simulink model "sampleModel1529"  (R2023a)
settings: Solver=VariableStepAuto  StartTime=0.0  StopTime=10.0  RelTol=1e-3
libraries: hdlsllib x6
settings Model: Creator=user1  LastModifiedBy=user1

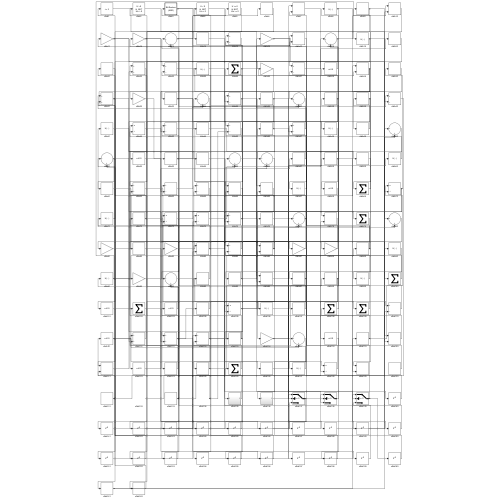
[thumbnail: Simulink's stored preview of the top-level diagram]
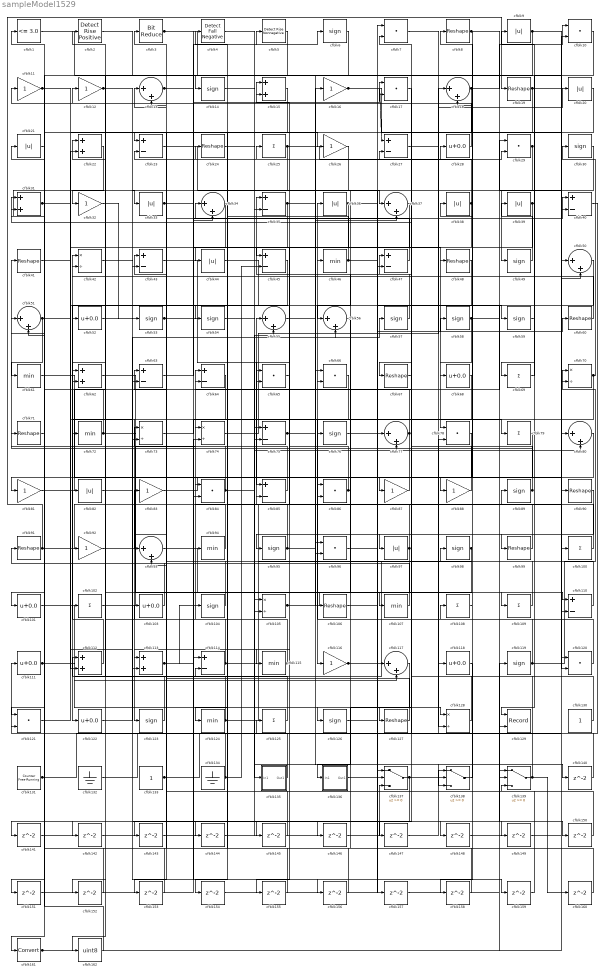
== system sampleModel1529 ==
  cfblk1 : hdlsllib/Logic and Bit Operations/Compare To Constant  relop=<=  const=3.0  OutDataTypeStr=boolean
  cfblk{7,10,17,29,65..66,78,84,86,96,120..121} (12 alike) : DotProduct  OutDataTypeStr=Inherit: Inherit via internal rule
  cfblk{25,69,79,100,102,108..109,125} (8 alike) : Sum  Inputs=+
  cfblk{28,52,68,101,103,111,118,122} (8 alike) : Bias  Bias=0.0  SaturateOnIntegerOverflow=off
  cfblk{6,14,30,49,53..54,57..59,76,89,95,98,104,119,123,126} (17 alike) : Signum
  cfblk{42,70,73..74,105,128} (6 alike) : Product  Inputs=*/  RndMeth=Zero  SaturateOnIntegerOverflow=on
  cfblk{8,19,24,41,48,60,67,71,90..91,99,106,127} (13 alike) : Reshape
  cfblk{46,61,72,94,107,115,124} (7 alike) : MinMax
  cfblk{11..12,16,26,32,81,83,87..88,92,116} (11 alike) : Gain
  cfblk{23,27,35,40,43,45,47,63..64,75,85,110,114} (13 alike) : Sum  Inputs=+-
  cfblk{15,22,31,62,112..113} (6 alike) : Sum
  cfblk{13,18,34,37,50..51,55..56,77,80,93,117} (12 alike) : Sum  Inputs=|++
  cfblk129 : Record  FileSettingsInternal="{\"entries\":[{\"content\":{\"excelSettings\":{\"content\":{},\"type\":\"Streamout.ExcelSettings\"}},\"type\":\"Streamout.FileSettingStorage\",\"uuid\":\"\"}],\"packageUris\":[\"http:\\/\\/schema.mathworks.com\\/mf0\\/streamout_blocks\\/R2020a\"],\"version\":\"1.0\"}"  Layout=[1 1]  SignalsInternal="{\"entries\":[{\"content\":{\"signals\":[{\"content\":{\"blockPath\":[],\"dimensions\":[1],\"domain\":\"\",\"lineColor\":\"#a2142f\",\"plots\":[1],\"port\":1,\"signalID\":1546,\"signalName\":\"XY Graph:1\"},\"type\":\"RecordBlkView.Signal\",\"uuid\":\"\"},{\"content\":{\"blockPath\":[],\"dimensions\":[1],\"domain\":\"\",\"lineColor\":\"#139fff\",\"plots\":[1],\"port\":2,\"signalID\":1549,\"signalName\":\"XY Graph:2\"},\"type\":\"RecordBlkView.Signal\",\"uuid\":\"\"}]},\"type\":\"RecordBlkView.InputSignals\",\"uuid\":\"\"}],\"packageUris\":[\"http:\\/\\/schema.mathworks.com\\/mf0\\/streamout_blocks\\/R2020a\"],\"version\":\"1.0\"}"  VisualizationBindings="{\"xyplotplugin\":{\"info\":[{\"series\":[{\"bindingParametersList\":[{\"parameter\":\"X-Axis\",\"signalID\":1546,\"signalName\":\"XY Graph:1\"},{\"parameter\":\"Y-Axis\",\"signalID\":1549,\"signalName\":\"XY Graph:2\"}],\"seriesID\":63561}],\"subplotID\":1}]}}"  CompatibilityTag=XY  st=-1
  cfblk130 : Constant  SampleTime=-1
  cfblk131 : hdlsllib/Sources/Counter Free-Running  NumBits=16  tsamp=-1
  cfblk132 : Ground
  cfblk133 : Constant  SampleTime=-1
  cfblk134 : Ground
  cfblk135 : Subsystem
      settings: LibrarySourceBlock=|
      | hdlsllib/Ports &
      | Subsystems/Subsystem
  cfblk136 : Subsystem
      settings: LibrarySourceBlock=|
      | hdlsllib/Ports &
      | Subsystems/Subsystem
  cfblk137 : Switch  SaturateOnIntegerOverflow=off  InputSameDT=off
  cfblk138 : Switch  SaturateOnIntegerOverflow=off  InputSameDT=off
  cfblk139 : Switch  SaturateOnIntegerOverflow=off  InputSameDT=off
  cfblk{140..160} (21 alike) : Delay  SampleTime=1
  cfblk161 : DataTypeConversion  SaturateOnIntegerOverflow=off  RndMeth=Floor
  cfblk162 : DataTypeConversion  OutDataTypeStr=uint8  SaturateOnIntegerOverflow=off  RndMeth=Floor
  cfblk2 : hdlsllib/Logic and Bit Operations/Detect Rise Positive  vinit=0  OutDataTypeStr=boolean
  cfblk{9,20..21,33,36,38..39,44,82,97} (10 alike) : Abs  SaturateOnIntegerOverflow=off
  cfblk3 : hdlsllib/Logic and Bit Operations/Bit Reduce  mode=AND
  cfblk4 : hdlsllib/Logic and Bit Operations/Detect Fall Negative  vinit=0  OutDataTypeStr=boolean
  cfblk5 : hdlsllib/Logic and Bit Operations/Detect Rise Nonnegative  vinit=0  OutDataTypeStr=boolean
  wires:
  cfblk115/1 -> cfblk64/1, cfblk113/1
  cfblk98/1 -> cfblk128/2, cfblk152/1
  cfblk38/1 -> cfblk78/1, cfblk112/2, cfblk4/1
  cfblk113/1 -> cfblk104/1, cfblk156/1
  cfblk87/1 -> cfblk81/1
  cfblk101/1 -> cfblk28/1
  cfblk29/1 -> cfblk49/1, cfblk105/2, cfblk47/2
  cfblk49/1 -> cfblk39/1
  cfblk100/1 -> cfblk55/1
  cfblk7/1 -> cfblk118/1
  cfblk43/1 -> cfblk85/1
  cfblk62/1 -> cfblk109/1
  cfblk58/1 -> cfblk68/1, cfblk150/1
  cfblk74/1 -> cfblk18/1
  cfblk10/1 -> cfblk69/1
  cfblk32/1 -> cfblk53/1
  cfblk85/1 -> cfblk41/1
  cfblk39/1 -> cfblk99/1, cfblk147/1
  cfblk68/1 -> cfblk116/1
  cfblk63/1 -> cfblk40/1
  cfblk119/1 -> cfblk70/1, cfblk47/1
  cfblk45/1 -> cfblk122/1
  cfblk31/1 -> cfblk73/2, cfblk151/1
  cfblk51/1 -> cfblk61/1, cfblk113/2
  cfblk71/1 -> cfblk33/1
  cfblk125/1 -> cfblk114/2
  cfblk112/1 -> cfblk42/1
  cfblk103/1 -> cfblk22/1
  cfblk99/1 -> cfblk34/1
  cfblk40/1 -> cfblk111/1
  cfblk70/1 -> cfblk123/1, cfblk30/1, cfblk96/2
  cfblk102/1 -> cfblk74/1
  cfblk95/1 -> cfblk85/2, cfblk57/1
  cfblk121/1 -> cfblk22/2
  cfblk20/1 -> cfblk62/1
  cfblk81/1 -> cfblk29/1
  cfblk59/1 -> cfblk129/1
  cfblk124/1 -> cfblk98/1, cfblk72/1
  cfblk91/1 -> cfblk19/1, cfblk86/2, cfblk92/1
  cfblk16/1 -> cfblk27/1, cfblk100/1
  cfblk123/1 -> cfblk112/1
  cfblk17/1 -> cfblk67/1
  cfblk105/1 -> cfblk110/1, cfblk17/1
  cfblk69/1 -> cfblk9/1
  cfblk114/1 -> cfblk50/1, cfblk62/2, cfblk138/3
  cfblk97/1 -> cfblk15/1, cfblk124/1
  cfblk66/1 -> cfblk102/1
  cfblk131/1 -> cfblk90/1, cfblk31/2
  cfblk92/1 -> cfblk83/1
  cfblk120/1 -> cfblk36/1
  cfblk6/1 -> cfblk52/1
  cfblk133/1 -> cfblk43/1, cfblk105/1, cfblk103/1
  cfblk96/1 -> cfblk7/1
  cfblk14/1 -> cfblk135/1(In1)
  cfblk28/1 -> cfblk12/1
  cfblk30/1 -> cfblk56/1
  cfblk127/1 -> cfblk63/1
  cfblk50/1 -> cfblk137/2
  cfblk83/1 -> cfblk87/1
  cfblk90/1 -> cfblk95/1
  cfblk109/1 -> cfblk76/1
  cfblk134/1 -> cfblk73/1, cfblk45/2
  cfblk73/1 -> cfblk79/1
  cfblk72/1 -> cfblk51/1, cfblk96/1
  cfblk44/1 -> cfblk129/2
  cfblk34/1 -> cfblk82/1
  cfblk47/1 -> cfblk3/1
  cfblk116/1 -> cfblk89/1, cfblk148/1
  cfblk60/1 -> cfblk42/2
  cfblk48/1 -> cfblk127/1
  cfblk46/1 -> cfblk117/1, cfblk23/2
  cfblk128/1 -> cfblk11/1
  cfblk126/1 -> cfblk58/1
  cfblk67/1 -> cfblk7/2
  cfblk9/1 -> cfblk120/1, cfblk101/1
  cfblk61/1 -> cfblk120/2
  cfblk8/1 -> cfblk40/2, cfblk88/1
  cfblk36/1 -> cfblk77/1, cfblk155/1
  cfblk57/1 -> cfblk35/1
  cfblk138/1 -> cfblk108/1
  cfblk37/1 -> cfblk65/1
  cfblk33/1 -> cfblk34/2, cfblk149/1
  cfblk22/1 -> cfblk32/1
  cfblk54/1 -> cfblk126/1
  cfblk117/1 -> cfblk136/1(In1)
  cfblk25/1 -> cfblk29/2, cfblk43/2
  cfblk18/1 -> cfblk121/1, cfblk10/1
  cfblk77/1 -> cfblk24/1, cfblk153/1
  cfblk86/1 -> cfblk15/2, cfblk46/1
  cfblk130/1 -> cfblk18/2
  cfblk132/1 -> cfblk78/2
  cfblk41/1 -> cfblk59/1
  cfblk1/1 -> cfblk66/1
  cfblk2/1 -> cfblk14/1
  cfblk13/1 -> cfblk5/1, cfblk17/2
  cfblk3/1 -> cfblk70/2, cfblk45/1
  cfblk19/1 -> cfblk80/1, cfblk44/1
  cfblk136/1(Out1) -> cfblk60/1
  cfblk108/1 -> cfblk38/1
  cfblk53/1 -> cfblk75/2, cfblk6/1
  cfblk24/1 -> cfblk35/2
  cfblk12/1 -> cfblk26/1, cfblk159/1
  cfblk78/1 -> cfblk115/1
  cfblk79/1 -> cfblk97/1
  cfblk94/1 -> cfblk84/1
  cfblk104/1 -> cfblk13/2
  cfblk23/1 -> cfblk37/1
  cfblk55/1 -> cfblk139/2
  cfblk93/1 -> cfblk107/1
  cfblk35/1 -> cfblk37/2, cfblk154/1
  cfblk26/1 -> cfblk63/2
  cfblk110/1 -> cfblk8/1
  cfblk27/1 -> cfblk20/1
  cfblk89/1 -> cfblk71/1, cfblk65/2
  cfblk107/1 -> cfblk91/1
  cfblk139/1 -> cfblk94/1, cfblk160/1
  cfblk52/1 -> cfblk86/1
  cfblk111/1 -> cfblk128/1, cfblk117/2
  cfblk4/1 -> cfblk48/1
  cfblk56/1 -> cfblk106/1
  cfblk64/1 -> cfblk93/1
  cfblk11/1 -> cfblk54/1, cfblk23/1
  cfblk84/1 -> cfblk2/1, cfblk80/2
  cfblk75/1 -> cfblk16/1, cfblk25/1
  cfblk88/1 -> cfblk31/1
  cfblk21/1 -> cfblk161/1
  cfblk122/1 -> cfblk56/2
  cfblk137/1 -> cfblk138/2, cfblk141/1
  cfblk135/1(Out1) -> cfblk125/1
  cfblk76/1 -> cfblk140/1
  cfblk140/1 -> cfblk27/2
  cfblk141/1 -> cfblk84/2
  cfblk80/1 -> cfblk142/1
  cfblk142/1 -> cfblk55/2
  cfblk15/1 -> cfblk143/1
  cfblk143/1 -> cfblk74/2
  cfblk42/1 -> cfblk144/1
  cfblk144/1 -> cfblk137/3
  cfblk65/1 -> cfblk145/1
  cfblk145/1 -> cfblk75/1
  cfblk82/1 -> cfblk146/1
  cfblk146/1 -> cfblk137/1
  cfblk147/1 -> cfblk138/1
  cfblk148/1 -> cfblk110/2
  cfblk149/1 -> cfblk50/2
  cfblk150/1 -> cfblk93/2
  cfblk151/1 -> cfblk114/1
  cfblk152/1 -> cfblk1/1
  cfblk153/1 -> cfblk121/2
  cfblk154/1 -> cfblk77/2
  cfblk155/1 -> cfblk51/2
  cfblk156/1 -> cfblk64/2
  cfblk106/1 -> cfblk157/1
  cfblk157/1 -> cfblk139/1
  cfblk118/1 -> cfblk158/1
  cfblk158/1 -> cfblk13/1
  cfblk159/1 -> cfblk139/3
  cfblk160/1 -> cfblk66/2
  cfblk161/1 -> cfblk10/2, cfblk119/1
  cfblk5/1 -> cfblk162/1
  cfblk162/1 -> cfblk21/1

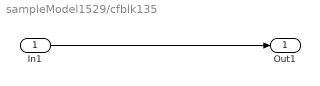
== system sampleModel1529/cfblk135 ==
  In1 : Inport
  Out1 : Outport
  wires:
  In1/1 -> Out1/1

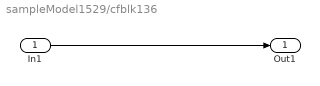
== system sampleModel1529/cfblk136 ==
  In1 : Inport
  Out1 : Outport
  wires:
  In1/1 -> Out1/1
